simulink model "Linearisation_Sim"  (R2018b)
settings: Solver=VariableStepAuto  StartTime=0.0  StopTime=30  FixedStep=1/60  RelTol=1e-5
undefined symbols (not defined in the file): d_initial, x_initial
settings Model: Creator=Naresh  LastModifiedBy=Naresh

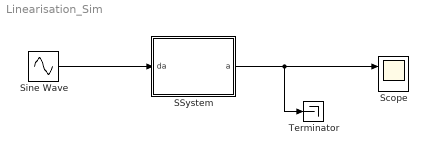
== system Linearisation_Sim ==
  SSystem : Subsystem
  Scope : Scope  NumInputPorts=2
  Sine Wave : Sin  Amplitude=3  Frequency=15  SampleTime=0
  Terminator : Terminator
  wires:
  SSystem/1(a) -> Terminator/1, Scope/1
  Sine Wave/1 -> SSystem/1(da)

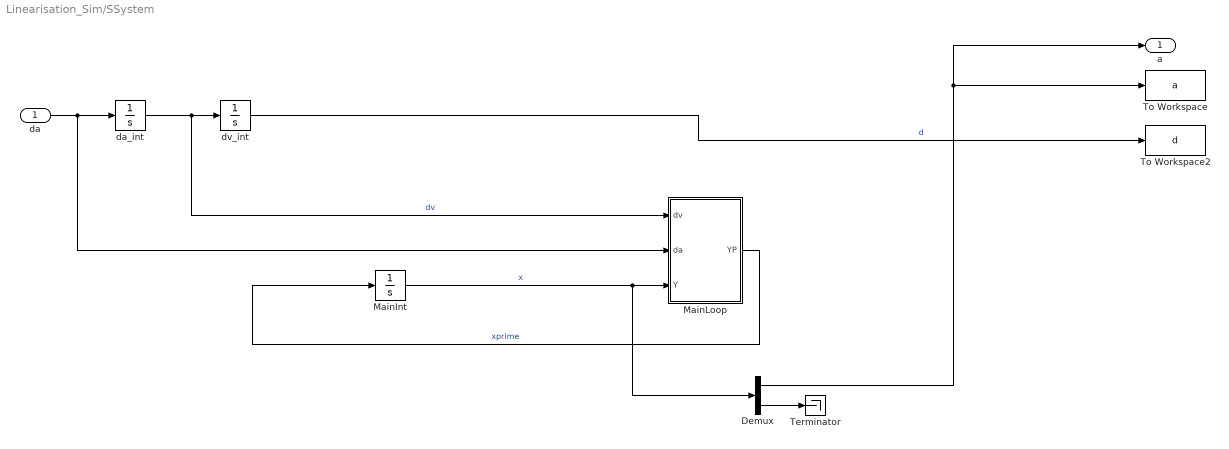
== system Linearisation_Sim/SSystem ==
  da : Inport
  Demux : Demux  Outputs=2
  MainInt : Integrator  InitialCondition=x_initial
  MainLoop : MATLAB Function  TreatAsAtomicUnit=on
  Terminator : Terminator
  To Workspace : ToWorkspace  VariableName=a  SaveFormat=Timeseries  SampleTime=-1
  To Workspace2 : ToWorkspace  VariableName=d  SaveFormat=Timeseries  SampleTime=-1
  da_int : Integrator  InitialCondition=d_initial(2)
  dv_int : Integrator  InitialCondition=d_initial(1)
  a : Outport
  wires:
  da/1 -> MainLoop/2(da), da_int/1
  MainInt/1 -> Demux/1, MainLoop/3(Y)  "x"
  da_int/1 -> MainLoop/1(dv), dv_int/1  "dv"
  MainLoop/1(YP) -> MainInt/1  "xprime"
  dv_int/1 -> To Workspace2/1  "d"
  Demux/2 -> Terminator/1
  Demux/1 -> a/1, To Workspace/1

== matlab function Linearisation_Sim/SSystem/MainLoop ==
  data: dv input; YP output; da input; Y input
function YP = MainLoop(dv,da,Y)
    g = 9.81;
    L = 10;
    m=2;
    lambda=1;

    YP = zeros(2,1);

    YP(1) = Y(2);
    YP(2) = (-L * lambda * Y(2) - dv * cos(Y(1)) * lambda - da * cos(Y(1)) * m - sin(Y(1)) * g * m) / L / m;

end
